simulink model "tanks1"  (R2016b)
settings: Solver=VariableStepAuto  StartTime=0.0  StopTime=10  RelTol=1e-3
libraries: simulink x1
settings Model: Creator=admin  LastModifiedBy=admin

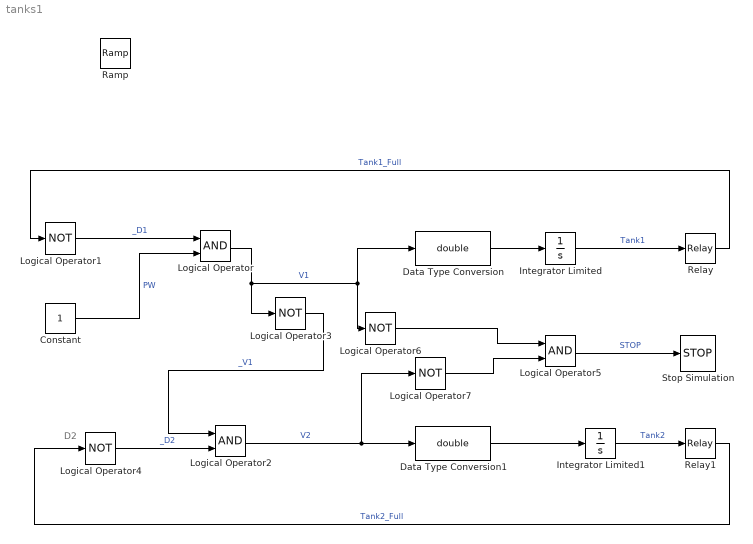
== system tanks1 ==
  note: D2
  Constant : Constant
  Data Type Conversion : DataTypeConversion  OutDataTypeStr=double  RndMeth=Round
  Data Type Conversion1 : DataTypeConversion  OutDataTypeStr=double  RndMeth=Round
  Integrator Limited : Integrator  LimitOutput=on  UpperSaturationLimit=1  LowerSaturationLimit=0
  Integrator Limited1 : Integrator  LimitOutput=on  UpperSaturationLimit=1  LowerSaturationLimit=0
  Logical Operator : Logic  AllPortsSameDT=off  OutDataTypeStr=boolean
  Logical Operator{1,3..4,6..7} (5 alike) : Logic  Operator=NOT  AllPortsSameDT=off  OutDataTypeStr=boolean
  Logical Operator2 : Logic  AllPortsSameDT=off  OutDataTypeStr=boolean
  Logical Operator5 : Logic  AllPortsSameDT=off  OutDataTypeStr=boolean
  Relay : Relay  OnSwitchValue=1  OffSwitchValue=0.99  OutDataTypeStr=int8
  Relay1 : Relay  OnSwitchValue=1  OffSwitchValue=0.99  OutDataTypeStr=int8
  Stop Simulation : Stop
  Ramp : simulink/Sources/Ramp  IOType=siggen  slope=1  start=0  X0=0
  wires:
  Logical Operator1/1 -> Logical Operator/1  "_D1"
  Logical Operator3/1 -> Logical Operator2/1  "_V1"
  Logical Operator2/1 -> Data Type Conversion1/1, Logical Operator7/1  "V2"
  Constant/1 -> Logical Operator/2  "PW"
  Logical Operator4/1 -> Logical Operator2/2  "_D2"
  Relay1/1 -> Logical Operator4/1  "Tank2_Full"
  Integrator Limited/1 -> Relay/1  "Tank1"
  Relay/1 -> Logical Operator1/1  "Tank1_Full"
  Integrator Limited1/1 -> Relay1/1  "Tank2"
  Logical Operator/1 -> Logical Operator3/1, Data Type Conversion/1, Logical Operator6/1  "V1"
  Data Type Conversion/1 -> Integrator Limited/1
  Data Type Conversion1/1 -> Integrator Limited1/1
  Logical Operator5/1 -> Stop Simulation/1  "STOP"
  Logical Operator6/1 -> Logical Operator5/1
  Logical Operator7/1 -> Logical Operator5/2
